simulink library "csu_mkf_multiplicative_update_lib"  (R2015b)
settings: Solver=ode45  SolverMode=SingleTasking  StartTime=0.0  StopTime=10.0  RelTol=1e-3
values from neighbouring files (symbols this model uses):
  mkf_null_quat = [ 0 0 0 1]    [csu_mkf_multiplicative_update_init.m]
  mkf_zero_gibbs = [ 0 0 0]    [csu_mkf_multiplicative_update_init.m]
undefined symbols (not defined in the file or in its folder): central_body_flattening, central_body_radius, central_body_rotation_rate, fcv_acquiring, fcv_initializing, ini_alt_wrt_meanrad, kfl_central_body_rotation_rate, mkf_cov_jam_index, mkf_cov_jam_matrix
libraries: util_quat_lib x10, util_common_lib x9, simulink x2, util_info_lib x2, util_fsw_frame_rotation_lib x2, util_frame_rotation_lib x1
settings Model: ExtModeAutoUpdateStatusClock=off  Creator=escrane  LastModifiedBy=Mark Agbayani
settings DataIOCC: SaveFormat=Array  SignalLoggingSaveFormat=ModelDataLogs
settings OptimizationCC: BlockReduction=off  BooleanDataType=off  ExpressionDepthLimit=2147483647
settings DebuggingCC: SaveWithParameterizedLinksMsg=none  UnderspecifiedInitializationDetection=Classic  MergeDetectMultiDrivingBlocksExec=none  SignalResolutionControl=TryResolveAllWithWarning  FcnCallInpInsideContextMsg=EnableAllAsWarning  StateNameClashWarn=warning  StrictBusMsg=Warning
settings HardwareCC: ProdBitPerPointer=32  ProdLargestAtomicFloat=None  ProdIntDivRoundTo=Undefined  ProdEndianess=Unspecified  ProdWordSize=32  ProdHWDeviceType=32-bit Generic  TargetUnknown=on
settings GRTTargetCC: GeneratePreprocessorConditionals=Disable all
settings ConfigComp: CovModelRefEnable=Off  CovSFcnEnable=off

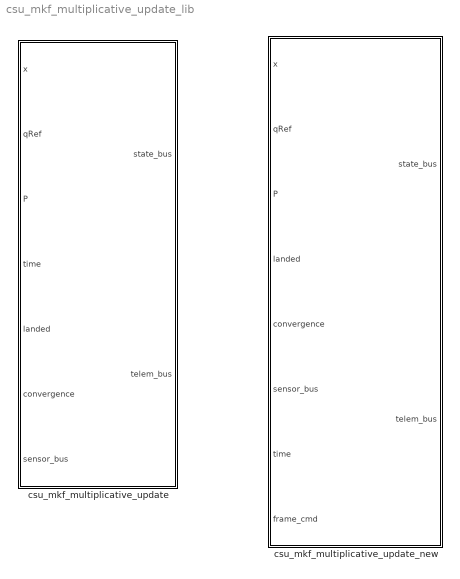
== system csu_mkf_multiplicative_update_lib ==
  csu_mkf_multiplicative_update : Subsystem
  csu_mkf_multiplicative_update_new : Subsystem

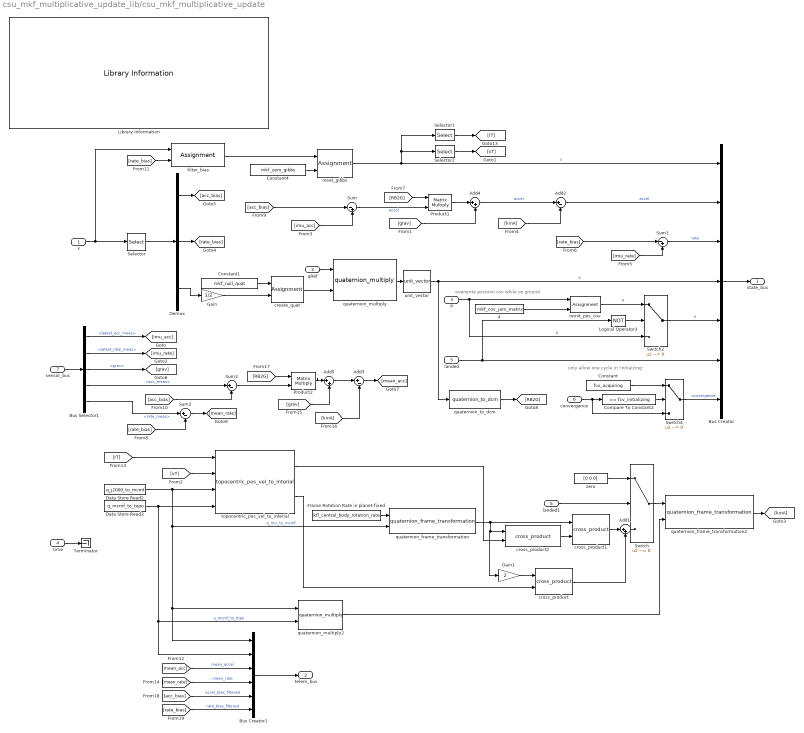
== system csu_mkf_multiplicative_update_lib/csu_mkf_multiplicative_update ==
  note: overwrite position cov while on ground
  note: only allow one cycle in 'initialzing'
  x : Inport
  qRef : Inport  Port=2
  P : Inport  Port=3
  time : Inport  Port=4
  landed : Inport  Port=5
  convergence : Inport  Port=6
  sensor_bus : Inport  Port=7
  "      4" : Constant  Value=mkf_cov_jam_matrix
  Add1 : Sum  Inputs=|++
  Add2 : Sum  Inputs=|+-
  Add3 : Sum  Inputs=|+-
  Add4 : Sum  Inputs=|++
  Add5 : Sum  Inputs=|++
  Bus Creator : BusCreator  Inputs=7
  Bus Creator1 : BusCreator  Inputs=6
  Bus Selector1 : BusSelector  OutputSignals=latest_acc_meas,latest_rate_meas,grav,acc_meas,rate_meas
  Compare To Constant2 : simulink/Logic and Bit Operations/Compare To Constant  relop===  const=fcv_initializing  OutDataTypeStr=boolean
  Constant : Constant  Value=fcv_acquiring  OutDataTypeStr=double
  Constant1 : Constant  Value=mkf_null_quat
  Constant4 : Constant  Value=mkf_zero_gibbs
  Data Store Read2 : DataStoreRead  DataStoreName=q_j2000_to_mcmf
  Data Store Read3 : DataStoreRead  DataStoreName=q_mcmf_to_topo
  Demux : Demux  Outputs=[3 3 3]
  Frame Rotation Rate in planet-fixed : Constant  Value=kfl_central_body_rotation_rate
  Gain : Gain  Gain=1/2
  Gain1 : Gain  Gain=2
  Library Information : util_info_lib/Library Information  owner='NONE'
  Logical Operator3 : Logic  Operator=NOT  AllPortsSameDT=off  OutDataTypeStr=boolean
  Product1 : Product  Multiplication=Matrix(*)  RndMeth=Zero
  Product2 : Product  Multiplication=Matrix(*)  RndMeth=Zero
  Selector : Selector  InputPortWidth=kfl_n_state  IndexOptions=Index vector (dialog)  Indices=mkf_selection_index  OutputSizes=1
  Selector1 : Selector  InputPortWidth=kfl_n_state  IndexOptions=Index vector (dialog)  Indices=kfl_pos_index  OutputSizes=1
  Selector2 : Selector  InputPortWidth=kfl_n_state  IndexOptions=Index vector (dialog)  Indices=kfl_vel_index  OutputSizes=1
  Sum : Sum  Inputs=|-+
  Sum1 : Sum  Inputs=|-+
  Sum2 : Sum  Inputs=|+-
  Sum3 : Sum  Inputs=|+-
  Switch : Switch  Criteria=u2 ~= 0
  Switch2 : Switch  Criteria=u2 ~= 0
  Switch4 : Switch  Criteria=u2 ~= 0  Threshold=0.5  InputSameDT=on
  Terminator : Terminator
  create_quat : Assignment  IndexOptions=Index vector (dialog)  Indices=[1 2 3]  OutputSizes=1
  cross_product : util_common_lib/cross_product  SystemSampleTime=-1
  cross_product1 : util_common_lib/cross_product  SystemSampleTime=-1
  cross_product2 : util_common_lib/cross_product  SystemSampleTime=-1
  filter_bias : Assignment  IndexOptions=Index vector (dialog)  Indices=kfl_gyro_bias_index  OutputSizes=1
  landed1 : InportShadow  Port=5
  quaternion_frame_transformation : util_quat_lib/quaternion_frame_transformation  SystemSampleTime=-1
  quaternion_frame_transformation2 : util_quat_lib/quaternion_frame_transformation  SystemSampleTime=-1
  quaternion_multiply : util_quat_lib/quaternion_multiply  SystemSampleTime=-1
  quaternion_multiply2 : util_quat_lib/quaternion_multiply  SystemSampleTime=-1
  quaternion_to_dcm : util_quat_lib/quaternion_to_dcm  SystemSampleTime=-1
  reinit_pos_cov : Assignment  NumberOfDimensions=2  IndexOptions=Index vector (dialog),Index vector (dialog)  Indices=mkf_cov_jam_index,mkf_cov_jam_index  OutputSizes=1,1
  reset_gibbs : Assignment  IndexOptions=Index vector (dialog)  Indices=kfl_gibbs_index  OutputSizes=1
  topocentric_pos_vel_to_interial : util_fsw_frame_rotation_lib/topocentric_pos_vel_to_interial  SystemSampleTime=-1
  unit_vector : util_common_lib/unit_vector  SystemSampleTime=-1
  zero : Constant  Value=[0 0 0]
  state_bus : Outport
  telem_bus : Outport  Port=2
  wires:
  [rate_bias] -> Bus Creator1/6  "rate_bias_filtered"
  [acc_bias] -> Bus Creator1/5  "accel_bias_filtered"
  Logical Operator3/1 -> Switch2/2
  Product1/1 -> Add4/1
  Add1/1 -> Switch/3
  landed1/1 -> Switch/2
  zero/1 -> Switch/1
  [grav] -> Add5/2
  Add3/1 -> [mean_acc]
  [RB2G] -> Product2/1
  Product2/1 -> Add5/1
  Add5/1 -> Add3/1
  [kinA] -> Add3/2
  Bus Creator1/1 -> telem_bus/1
  [mean_acc] -> Bus Creator1/3  "mean_accel"
  [mean_rate] -> Bus Creator1/4  "mean_rate"
  [rate_bias] -> filter_bias/2
  Sum3/1 -> Product2/2
  [acc_bias] -> Sum3/2
  [acc_bias] -> Sum/1
  Demux/1 -> [acc_bias]
  [rate_bias] -> Sum2/2
  Sum2/1 -> [mean_rate]
  [rate_bias] -> Sum1/1
  Bus Selector1/2 -> [imu_rate]  "<latest_rate_meas>"
  Bus Selector1/5 -> Sum2/1  "<rate_meas>"
  Bus Selector1/4 -> Sum3/1  "<acc_meas>"
  Bus Selector1/3 -> [grav]  "<grav>"
  Constant/1 -> Switch4/1
  Compare To Constant2/1 -> Switch4/2
  convergence/1 -> Compare To Constant2/1, Switch4/3
  quaternion_multiply2/1 -> quaternion_frame_transformation2/2
  quaternion_frame_transformation2/1 -> [kinA]
  Switch/1 -> quaternion_frame_transformation2/1
  topocentric_pos_vel_to_interial/1 -> cross_product2/2
  Switch4/1 -> Bus Creator/7  "convergence"
  "      4"/1 -> reinit_pos_cov/2
  Switch2/1 -> Bus Creator/5  "P"
  reinit_pos_cov/1 -> Switch2/1  "P"
  landed/1 -> Logical Operator3/1, Bus Creator/6
  P/1 -> reinit_pos_cov/1, Switch2/3  "P"
  filter_bias/1 -> reset_gibbs/1
  Demux/2 -> [rate_bias]
  x/1 -> Selector/1, filter_bias/1
  create_quat/1 -> quaternion_multiply/2
  qRef/1 -> quaternion_multiply/1
  Demux/3 -> Gain/1
  Bus Creator/1 -> state_bus/1
  time/1 -> Terminator/1
  Selector/1 -> Demux/1
  sensor_bus/1 -> Bus Selector1/1
  Bus Selector1/1 -> [imu_acc]  "<latest_acc_meas>"
  [imu_acc] -> Sum/2
  [imu_rate] -> Sum1/2
  reset_gibbs/1 -> Selector2/1, Selector1/1, Bus Creator/1  "x"
  Sum1/1 -> Bus Creator/3  "rate"
  Constant4/1 -> reset_gibbs/2
  quaternion_multiply/1 -> unit_vector/1
  Constant1/1 -> create_quat/1
  Gain/1 -> create_quat/2
  unit_vector/1 -> quaternion_to_dcm/1, Bus Creator/4  "q"
  Sum/1 -> Product1/2  "accel"
  quaternion_to_dcm/1 -> [RB2G]
  [RB2G] -> Product1/1
  [grav] -> Add4/2
  Frame Rotation Rate in planet-fixed/1 -> quaternion_frame_transformation/1
  Data Store Read3/1 -> quaternion_multiply2/2, Bus Creator1/2, topocentric_pos_vel_to_interial/4  "q_mcmf_to_topo"
  Selector1/1 -> [rT]
  Selector2/1 -> [vT]
  quaternion_frame_transformation/1 -> cross_product2/1, Gain1/1, cross_product1/1
  Gain1/1 -> cross_product/1
  cross_product2/1 -> cross_product1/2
  cross_product1/1 -> Add1/1
  Add4/1 -> Add2/1  "accel"
  Add2/1 -> Bus Creator/2  "accel"
  [kinA] -> Add2/2
  [vT] -> topocentric_pos_vel_to_interial/2
  [rT] -> topocentric_pos_vel_to_interial/1
  Data Store Read2/1 -> quaternion_frame_transformation/2, Bus Creator1/1, quaternion_multiply2/1, topocentric_pos_vel_to_interial/3  "q_mci_to_mcmf"
  topocentric_pos_vel_to_interial/2 -> cross_product/2
  cross_product/1 -> Add1/2

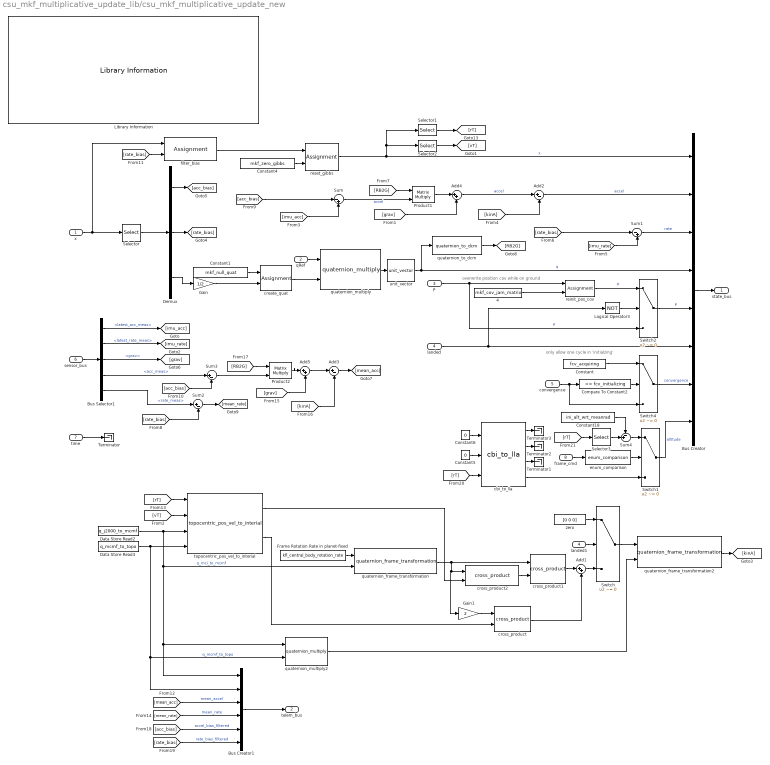
== system csu_mkf_multiplicative_update_lib/csu_mkf_multiplicative_update_new ==
  note: only allow one cycle in 'initialzing'
  note: overwrite position cov while on ground
  x : Inport
  qRef : Inport  Port=2
  P : Inport  Port=3
  landed : Inport  Port=4
  convergence : Inport  Port=5
  sensor_bus : Inport  Port=6
  time : Inport  Port=7
  frame_cmd : Inport  Port=8
  "      4" : Constant  Value=mkf_cov_jam_matrix
  Add1 : Sum  Inputs=|++
  Add2 : Sum  Inputs=|+-
  Add3 : Sum  Inputs=|+-
  Add4 : Sum  Inputs=|++
  Add5 : Sum  Inputs=|++
  Bus Creator : BusCreator  Inputs=8
  Bus Creator1 : BusCreator  Inputs=6
  Bus Selector1 : BusSelector  OutputSignals=latest_acc_meas,latest_rate_meas,grav,acc_meas,rate_meas
  Compare To Constant2 : simulink/Logic and Bit Operations/Compare To Constant  relop===  const=fcv_initializing  OutDataTypeStr=boolean
  Constant : Constant  Value=fcv_acquiring  OutDataTypeStr=double
  Constant1 : Constant  Value=mkf_null_quat
  Constant18 : Constant  Value=ini_alt_wrt_meanrad
  Constant4 : Constant  Value=mkf_zero_gibbs
  Constant5 : Constant  Value=0
  Constant6 : Constant  Value=0
  Data Store Read2 : DataStoreRead  DataStoreName=q_j2000_to_mcmf
  Data Store Read3 : DataStoreRead  DataStoreName=q_mcmf_to_topo
  Demux : Demux  Outputs=[3 3 3]
  Frame Rotation Rate in planet-fixed : Constant  Value=kfl_central_body_rotation_rate
  Gain : Gain  Gain=1/2
  Gain1 : Gain  Gain=2
  Library Information : util_info_lib/Library Information  owner='NONE'
  Logical Operator3 : Logic  Operator=NOT  AllPortsSameDT=off  OutDataTypeStr=boolean
  Product1 : Product  Multiplication=Matrix(*)  RndMeth=Zero
  Product2 : Product  Multiplication=Matrix(*)  RndMeth=Zero
  Selector : Selector  InputPortWidth=kfl_n_state  IndexOptions=Index vector (dialog)  Indices=mkf_selection_index  OutputSizes=1
  Selector1 : Selector  InputPortWidth=kfl_n_state  IndexOptions=Index vector (dialog)  Indices=kfl_pos_index  OutputSizes=1
  Selector2 : Selector  InputPortWidth=kfl_n_state  IndexOptions=Index vector (dialog)  Indices=kfl_vel_index  OutputSizes=1
  Selector3 : Selector  InputPortWidth=3  IndexOptions=Index vector (dialog)  Indices=[3]  OutputSizes=1
  Sum : Sum  Inputs=|-+
  Sum1 : Sum  Inputs=|-+
  Sum2 : Sum  Inputs=|+-
  Sum3 : Sum  Inputs=|+-
  Sum4 : Sum  Inputs=-+|
  Switch : Switch  Criteria=u2 ~= 0
  Switch1 : Switch  Criteria=u2 ~= 0  Threshold=0.5  InputSameDT=on
  Switch2 : Switch  Criteria=u2 ~= 0
  Switch4 : Switch  Criteria=u2 ~= 0  Threshold=0.5  InputSameDT=on
  Terminator{,1..3} (4 alike) : Terminator
  cbi_to_lla : util_frame_rotation_lib/cbi_to_lla  a=central_body_radius  b=central_body_radius*(1-central_body_flattening)  omega=central_body_rotation_rate(3)
  create_quat : Assignment  IndexOptions=Index vector (dialog)  Indices=[1 2 3]  OutputSizes=1
  cross_product : util_common_lib/cross_product  SystemSampleTime=-1
  cross_product1 : util_common_lib/cross_product  SystemSampleTime=-1
  cross_product2 : util_common_lib/cross_product  SystemSampleTime=-1
  enum_comparison : util_common_lib/enum_comparison  comparison_type===
  filter_bias : Assignment  IndexOptions=Index vector (dialog)  Indices=kfl_gyro_bias_index  OutputSizes=1
  landed1 : InportShadow  Port=4
  quaternion_frame_transformation : util_quat_lib/quaternion_frame_transformation  SystemSampleTime=-1
  quaternion_frame_transformation2 : util_quat_lib/quaternion_frame_transformation  SystemSampleTime=-1
  quaternion_multiply : util_quat_lib/quaternion_multiply  SystemSampleTime=-1
  quaternion_multiply2 : util_quat_lib/quaternion_multiply  SystemSampleTime=-1
  quaternion_to_dcm : util_quat_lib/quaternion_to_dcm  SystemSampleTime=-1
  reinit_pos_cov : Assignment  NumberOfDimensions=2  IndexOptions=Index vector (dialog),Index vector (dialog)  Indices=mkf_cov_jam_index,mkf_cov_jam_index  OutputSizes=1,1
  reset_gibbs : Assignment  IndexOptions=Index vector (dialog)  Indices=kfl_gibbs_index  OutputSizes=1
  topocentric_pos_vel_to_interial : util_fsw_frame_rotation_lib/topocentric_pos_vel_to_interial  SystemSampleTime=-1
  unit_vector : util_common_lib/unit_vector  SystemSampleTime=-1
  zero : Constant  Value=[0 0 0]
  state_bus : Outport
  telem_bus : Outport  Port=2
  wires:
  Constant18/1 -> Sum4/1
  Sum4/1 -> Switch1/1
  Selector3/1 -> Sum4/2
  time/1 -> Terminator/1
  [rT] -> cbi_to_lla/3
  [rT] -> Selector3/1
  enum_comparison/1 -> Switch1/2
  frame_cmd/1 -> enum_comparison/1
  cross_product/1 -> Add1/2
  topocentric_pos_vel_to_interial/2 -> cross_product/2
  Data Store Read2/1 -> topocentric_pos_vel_to_interial/3, quaternion_multiply2/1, Bus Creator1/1, quaternion_frame_transformation/2  "q_mci_to_mcmf"
  [rT] -> topocentric_pos_vel_to_interial/1
  [vT] -> topocentric_pos_vel_to_interial/2
  [kinA] -> Add2/2
  Add2/1 -> Bus Creator/2  "accel"
  Add4/1 -> Add2/1  "accel"
  cross_product1/1 -> Add1/1
  cross_product2/1 -> cross_product1/2
  Gain1/1 -> cross_product/1
  quaternion_frame_transformation/1 -> cross_product1/1, Gain1/1, cross_product2/1
  Selector2/1 -> [vT]
  Selector1/1 -> [rT]
  Data Store Read3/1 -> topocentric_pos_vel_to_interial/4, Bus Creator1/2, quaternion_multiply2/2  "q_mcmf_to_topo"
  Frame Rotation Rate in planet-fixed/1 -> quaternion_frame_transformation/1
  [grav] -> Add4/2
  [RB2G] -> Product1/1
  quaternion_to_dcm/1 -> [RB2G]
  Sum/1 -> Product1/2  "accel"
  unit_vector/1 -> quaternion_to_dcm/1, Bus Creator/4  "q"
  Gain/1 -> create_quat/2
  Constant1/1 -> create_quat/1
  quaternion_multiply/1 -> unit_vector/1
  Constant4/1 -> reset_gibbs/2
  Sum1/1 -> Bus Creator/3  "rate"
  reset_gibbs/1 -> Bus Creator/1, Selector1/1, Selector2/1  "x"
  [imu_rate] -> Sum1/2
  [imu_acc] -> Sum/2
  Bus Selector1/1 -> [imu_acc]  "<latest_acc_meas>"
  sensor_bus/1 -> Bus Selector1/1
  Selector/1 -> Demux/1
  Bus Creator/1 -> state_bus/1
  Demux/3 -> Gain/1
  qRef/1 -> quaternion_multiply/1
  create_quat/1 -> quaternion_multiply/2
  x/1 -> filter_bias/1, Selector/1
  Demux/2 -> [rate_bias]
  filter_bias/1 -> reset_gibbs/1
  P/1 -> Switch2/3, reinit_pos_cov/1  "P"
  landed/1 -> Logical Operator3/1, Bus Creator/6
  reinit_pos_cov/1 -> Switch2/1  "P"
  Switch2/1 -> Bus Creator/5  "P"
  "      4"/1 -> reinit_pos_cov/2
  Switch4/1 -> Bus Creator/7  "convergence"
  topocentric_pos_vel_to_interial/1 -> cross_product2/2
  Switch/1 -> quaternion_frame_transformation2/1
  quaternion_frame_transformation2/1 -> [kinA]
  quaternion_multiply2/1 -> quaternion_frame_transformation2/2
  convergence/1 -> Switch4/3, Compare To Constant2/1
  Compare To Constant2/1 -> Switch4/2
  Constant/1 -> Switch4/1
  Bus Selector1/3 -> [grav]  "<grav>"
  Bus Selector1/4 -> Sum3/1  "<acc_meas>"
  Bus Selector1/5 -> Sum2/1  "<rate_meas>"
  Bus Selector1/2 -> [imu_rate]  "<latest_rate_meas>"
  [rate_bias] -> Sum1/1
  Sum2/1 -> [mean_rate]
  [rate_bias] -> Sum2/2
  Demux/1 -> [acc_bias]
  [acc_bias] -> Sum/1
  [acc_bias] -> Sum3/2
  Sum3/1 -> Product2/2
  [rate_bias] -> filter_bias/2
  [mean_rate] -> Bus Creator1/4  "mean_rate"
  [mean_acc] -> Bus Creator1/3  "mean_accel"
  Bus Creator1/1 -> telem_bus/1
  [kinA] -> Add3/2
  Add5/1 -> Add3/1
  Product2/1 -> Add5/1
  [RB2G] -> Product2/1
  Add3/1 -> [mean_acc]
  [grav] -> Add5/2
  zero/1 -> Switch/1
  landed1/1 -> Switch/2
  Add1/1 -> Switch/3
  Product1/1 -> Add4/1
  Logical Operator3/1 -> Switch2/2
  [acc_bias] -> Bus Creator1/5  "accel_bias_filtered"
  [rate_bias] -> Bus Creator1/6  "rate_bias_filtered"
  Switch1/1 -> Bus Creator/8  "altitude"
  Constant5/1 -> cbi_to_lla/2
  Constant6/1 -> cbi_to_lla/1
  cbi_to_lla/3 -> Terminator1/1
  cbi_to_lla/2 -> Terminator2/1
  cbi_to_lla/1 -> Terminator3/1
  cbi_to_lla/4 -> Switch1/3
